simulink model "FYP_Flywheel_Stage4_v2_StableClosedLoop"  (R2024a)
settings: Solver=ode45  StartTime=0.0  StopTime=18  RelTol=1e-3
values from neighbouring files (symbols this model uses):
  B = 1.0e-3    (= 0.001)    [FYP_Flywheel_Stage2_build.m]    (also in FYP_Flywheel_Stage3_DCServo_build.m; FYP_Flywheel_Stage4_v2_StableClosedLoop_build.m; FYP_Flywheel_Stage5_COMPLETE_v2.m)
  Imax = 18    [FYP_Flywheel_Stage4_v2_StableClosedLoop_build.m]    (also in FYP_Flywheel_Stage5_COMPLETE_v2.m = 20)
  J_total = Jm + Jf    (= 0.51)    [FYP_Flywheel_Stage3_DCServo_build.m]    (also in FYP_Flywheel_Stage4_v2_StableClosedLoop_build.m; FYP_Flywheel_Stage5_COMPLETE_v2.m)
  Jf = 0.50    (= 0.5)    [FYP_Flywheel_Stage3_DCServo_build.m]    (also in FYP_Flywheel_Stage4_v2_StableClosedLoop_build.m; FYP_Flywheel_Stage5_COMPLETE_v2.m)
  Ke = 0.05    [FYP_Flywheel_Stage3_DCServo_build.m]    (also in FYP_Flywheel_Stage4_v2_StableClosedLoop_build.m; FYP_Flywheel_Stage5_COMPLETE_v2.m)
  Kp_current = 1.0    (= 1)    [FYP_Flywheel_Stage4_v2_StableClosedLoop_build.m]    (also in FYP_Flywheel_Stage5_COMPLETE_v2.m)
  Kp_speed = 2.0    (= 2)    [FYP_Flywheel_Stage4_v2_StableClosedLoop_build.m]
  Kt = 0.05    [FYP_Flywheel_Stage3_DCServo_build.m]    (also in FYP_Flywheel_Stage4_v2_StableClosedLoop_build.m; FYP_Flywheel_Stage5_COMPLETE_v2.m)
  L = 0.02    [FYP_Flywheel_Stage3_DCServo_build.m]    (also in FYP_Flywheel_Stage4_v2_StableClosedLoop_build.m; FYP_Flywheel_Stage5_COMPLETE_v2.m)
  omega0 = 2*pi*n0/60    (= 314.159265359)    [FYP_Flywheel_Stage1_build.m]    (also in FYP_Flywheel_Stage2_build.m; FYP_Flywheel_Stage3_DCServo_build.m; FYP_Flywheel_Stage4_v2_StableClosedLoop_build.m; FYP_Flywheel_Stage5_COMPLETE_v2.m)
  R = 0.8    [FYP_Flywheel_Stage3_DCServo_build.m]    (also in FYP_Flywheel_Stage4_v2_StableClosedLoop_build.m; FYP_Flywheel_Stage5_COMPLETE_v2.m)
  Tc = 0.05    [FYP_Flywheel_Stage2_build.m]    (also in FYP_Flywheel_Stage3_DCServo_build.m; FYP_Flywheel_Stage4_v2_StableClosedLoop_build.m; FYP_Flywheel_Stage5_COMPLETE_v2.m)
  Vmax = 60    [FYP_Flywheel_Stage4_v2_StableClosedLoop_build.m]    (also in FYP_Flywheel_Stage5_COMPLETE_v2.m)
settings Model: Creator=cheng  LastModifiedBy=cheng

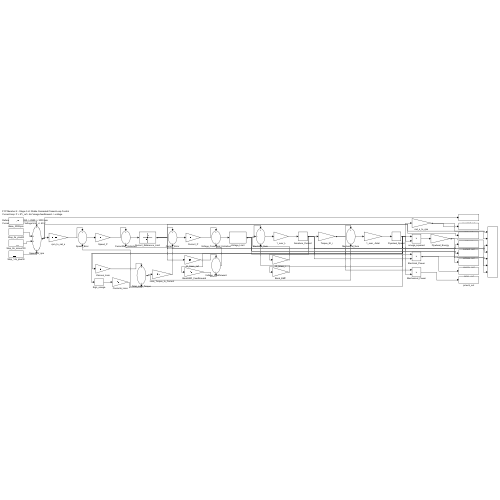
[thumbnail: Simulink's stored preview of the top-level diagram]
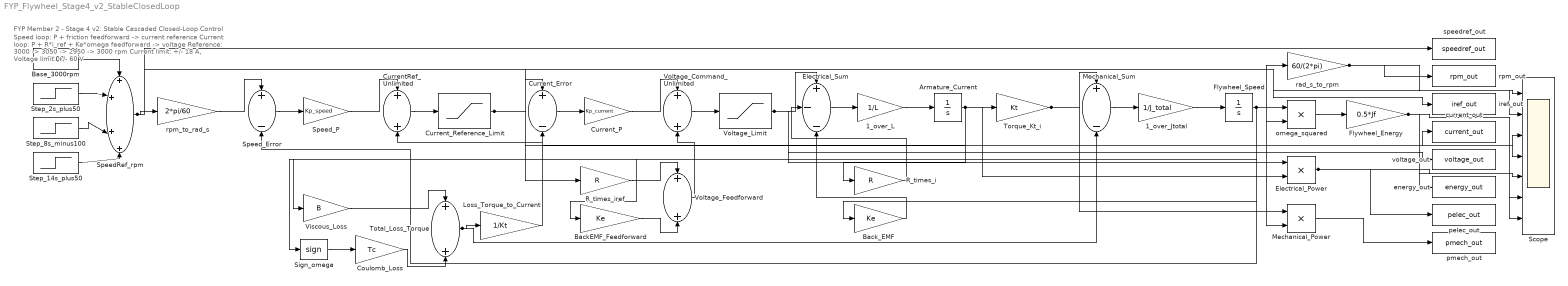
== system FYP_Flywheel_Stage4_v2_StableClosedLoop ==
  note: FYP Member 2 - Stage 4 v2: Stable Cascaded Closed-Loop Control
  note: Speed loop: P + friction feedforward -> current reference
      | Current loop: P + R*i_ref + Ke*omega feedforward -> voltage
      |
      | Reference: 3000 -> 3050 -> 2950 -> 3000 rpm
      | Current limit: +/- 18 A, Voltage limit: +/- 60 V
  1_over_Jtotal : Gain  Gain=1/J_total
  1_over_L : Gain  Gain=1/L
  Armature_Current : Integrator
  BackEMF_Feedforward : Gain  Gain=Ke
  Back_EMF : Gain  Gain=Ke
  Base_3000rpm : Constant  Value=3000
  Coulomb_Loss : Gain  Gain=Tc
  CurrentRef_Unlimited : Sum
  Current_Error : Sum  Inputs=+-
  Current_P : Gain  Gain=Kp_current
  Current_Reference_Limit : Saturate  UpperLimit=Imax  LowerLimit=-Imax
  Electrical_Power : Product  Inputs=**
  Electrical_Sum : Sum  Inputs=+--
  Flywheel_Energy : Gain  Gain=0.5*Jf
  Flywheel_Speed : Integrator  InitialCondition=omega0
  Loss_Torque_to_Current : Gain  Gain=1/Kt
  Mechanical_Power : Product  Inputs=**
  Mechanical_Sum : Sum  Inputs=+-
  R_times_i : Gain  Gain=R
  R_times_iref : Gain  Gain=R
  Scope : Scope  NumInputPorts=7
  Sign_omega : Signum
  SpeedRef_rpm : Sum  Inputs=++++
  Speed_Error : Sum  Inputs=+-
  Speed_P : Gain  Gain=Kp_speed
  Step_14s_plus50 : Step  Time=14  After=50  SampleTime=0
  Step_2s_plus50 : Step  Time=2  After=50  SampleTime=0
  Step_8s_minus100 : Step  Time=8  After=-100  SampleTime=0
  Torque_Kt_i : Gain  Gain=Kt
  Total_Loss_Torque : Sum
  Viscous_Loss : Gain  Gain=B
  Voltage_Command_Unlimited : Sum
  Voltage_Feedforward : Sum
  Voltage_Limit : Saturate  UpperLimit=Vmax  LowerLimit=-Vmax
  current_out : ToWorkspace  VariableName=current_out  SaveFormat=Timeseries  SampleTime=-1
  energy_out : ToWorkspace  VariableName=energy_out  SaveFormat=Timeseries  SampleTime=-1
  iref_out : ToWorkspace  VariableName=iref_out  SaveFormat=Timeseries  SampleTime=-1
  omega_squared : Product  Inputs=**
  pelec_out : ToWorkspace  VariableName=pelec_out  SaveFormat=Timeseries  SampleTime=-1
  pmech_out : ToWorkspace  VariableName=pmech_out  SaveFormat=Timeseries  SampleTime=-1
  rad_s_to_rpm : Gain  Gain=60/(2*pi)
  rpm_out : ToWorkspace  VariableName=rpm_out  SaveFormat=Timeseries  SampleTime=-1
  rpm_to_rad_s : Gain  Gain=2*pi/60
  speedref_out : ToWorkspace  VariableName=speedref_out  SaveFormat=Timeseries  SampleTime=-1
  voltage_out : ToWorkspace  VariableName=voltage_out  SaveFormat=Timeseries  SampleTime=-1
  wires:
  Base_3000rpm/1 -> SpeedRef_rpm/1
  Step_2s_plus50/1 -> SpeedRef_rpm/2
  Step_8s_minus100/1 -> SpeedRef_rpm/3
  Step_14s_plus50/1 -> SpeedRef_rpm/4
  SpeedRef_rpm/1 -> rpm_to_rad_s/1, speedref_out/1, Scope/1
  rpm_to_rad_s/1 -> Speed_Error/1
  Speed_Error/1 -> Speed_P/1
  Speed_P/1 -> CurrentRef_Unlimited/1
  Loss_Torque_to_Current/1 -> CurrentRef_Unlimited/2
  CurrentRef_Unlimited/1 -> Current_Reference_Limit/1
  Current_Reference_Limit/1 -> Current_Error/1, R_times_iref/1, iref_out/1, Scope/3
  Current_Error/1 -> Current_P/1
  R_times_iref/1 -> Voltage_Feedforward/1
  BackEMF_Feedforward/1 -> Voltage_Feedforward/2
  Current_P/1 -> Voltage_Command_Unlimited/1
  Voltage_Feedforward/1 -> Voltage_Command_Unlimited/2
  Voltage_Command_Unlimited/1 -> Voltage_Limit/1
  Voltage_Limit/1 -> Electrical_Sum/1, Electrical_Power/1, voltage_out/1, Scope/5
  Electrical_Sum/1 -> 1_over_L/1
  1_over_L/1 -> Armature_Current/1
  Armature_Current/1 -> Current_Error/2, R_times_i/1, Torque_Kt_i/1, Electrical_Power/2, current_out/1, Scope/4
  R_times_i/1 -> Electrical_Sum/2
  Torque_Kt_i/1 -> Mechanical_Sum/1, Mechanical_Power/1
  Total_Loss_Torque/1 -> Mechanical_Sum/2, Loss_Torque_to_Current/1
  Mechanical_Sum/1 -> 1_over_Jtotal/1
  1_over_Jtotal/1 -> Flywheel_Speed/1
  Flywheel_Speed/1 -> Speed_Error/2, Viscous_Loss/1, Sign_omega/1, Back_EMF/1, BackEMF_Feedforward/1, rad_s_to_rpm/1, omega_squared/1, omega_squared/2, Mechanical_Power/2
  Viscous_Loss/1 -> Total_Loss_Torque/1
  Sign_omega/1 -> Coulomb_Loss/1
  Coulomb_Loss/1 -> Total_Loss_Torque/2
  Back_EMF/1 -> Electrical_Sum/3
  omega_squared/1 -> Flywheel_Energy/1
  rad_s_to_rpm/1 -> rpm_out/1, Scope/2
  Flywheel_Energy/1 -> energy_out/1, Scope/6
  Electrical_Power/1 -> pelec_out/1, Scope/7
  Mechanical_Power/1 -> pmech_out/1
